simulink model "Proj2_P4_2"  (Simulink 8.6)
settings: Solver=ode45  StartTime=0.0  StopTime=10  MaxStep=0.001  RelTol=1e-3
values from neighbouring files (symbols this model uses):
  fl_rd_0 = fl_rd_rated    [Proj2_IM_IC_rated.m]    (also in Proj2_P1_calc.m = eps)
  fl_rd_0_est2 = fl_rd_rated_est2    [Proj2_P4_S2.m]    (also in Proj2_P4_calc2.m = fl_rd_0; Proj2_P4_calc3.m = fl_rd_0)
  fl_rd_0_est3 = fl_rd_rated    [Proj2_P4_S3.m]    (also in Proj2_P4_calc2.m = fl_rd_0; Proj2_P4_calc3.m = fl_rd_0)
  fl_sd_0 = fl_sd_rated    [Proj2_IM_IC_rated.m]    (also in Proj2_P1_calc.m = 0)
  fl_sq_0 = fl_sq_rated    [Proj2_IM_IC_rated.m]    (also in Proj2_P1_calc.m = 0)
  Isd_rated = real(Is_rated)    [Proj2_IM_IC_rated.m]
  Isd_rated_est2 = real(Is_rated_est2)    [Proj2_P4_S2.m]    (also in Proj2_P4_calc2.m = Isd_rated)
  Isd_rated_est3 = real(Is_rated_est3)    [Proj2_P4_S3.m]    (also in Proj2_P4_calc2.m = Isd_rated)
  Isq_0 = Isq_rated    [Proj2_IM_IC_rated.m]
  Isq_0_est2 = Isq_rated_est2    [Proj2_P4_S2.m]    (also in Proj2_P4_calc2.m = Isq_0; Proj2_P4_calc3.m = Isq_0)
  Isq_0_est3 = Isq_rated_est3    [Proj2_P4_S3.m]    (also in Proj2_P4_calc2.m = Isq_0; Proj2_P4_calc3.m = Isq_0)
  J_eq = 75    [Proj2_IM_parameters.m]
  Ki_i = w_c_i*sqrt(R_s^2+(w_c_i*L_s*sigma)^2) / sqrt(1+wc_Kp_by_Ki_for_i^2)    [Proj2_IM_IC_rated.m]
  Ki_i_est3 = w_c_i*sqrt(R_s^2+(w_c_i*L_s*sigma_est3)^2) / sqrt(1+wc_Kp_by_Ki_for_i_est3^2)    [Proj2_P4_S3.m]    (also in Proj2_P4_calc2.m = Ki_i)
  Ki_s = w_c_s^2*J_eq/(k*sqrt(1+tan(PM_s)^2))    [Proj2_IM_IC_rated.m]
  Ki_s_est2 = w_c_s^2*J_eq/(k_est2*sqrt(1+tan(PM_s)^2))    [Proj2_P4_S2.m]    (also in Proj2_P4_calc2.m = Ki_s)
  Ki_s_est3 = w_c_s^2*J_eq/(k_est3*sqrt(1+tan(PM_s)^2))    [Proj2_P4_S3.m]    (also in Proj2_P4_calc2.m = Ki_s)
  Kp_i = Ki_i * wc_Kp_by_Ki_for_i / w_c_i    [Proj2_IM_IC_rated.m]
  Kp_i_est3 = Ki_i_est3 * wc_Kp_by_Ki_for_i_est3 / w_c_i    [Proj2_P4_S3.m]    (also in Proj2_P4_calc2.m = Kp_i)
  Kp_s = Ki_s * wc_Kp_by_Ki_for_s / w_c_s    [Proj2_IM_IC_rated.m]
  Kp_s_est2 = Ki_s_est2 * wc_Kp_by_Ki_for_s / w_c_s    [Proj2_P4_S2.m]    (also in Proj2_P4_calc2.m = Kp_s)
  Kp_s_est3 = Ki_s_est3 * wc_Kp_by_Ki_for_s / w_c_s    [Proj2_P4_S3.m]    (also in Proj2_P4_calc2.m = Kp_s)
  L_m = X_m /w_syn    (= 0.00152788745368)    [Proj2_IM_parameters.m]
  L_r = L_lr+L_m    (= 0.00161011750761)    [Proj2_IM_parameters.m]
  L_r_est3 = L_lr_est3 + L_m    [Proj2_P4_S3.m]
  L_s = L_ls+L_m    (= 0.00161807525477)    [Proj2_IM_parameters.m]
  p = 6    [Proj2_IM_parameters.m]
  R_s = 1.4*10^-3    (= 0.0014)    [Proj2_IM_parameters.m]
  T_L_rated = T_em_rated    [Proj2_IM_parameters.m]
  tau_r = L_r/R_r    (= 1.62474016914)    [Proj2_IM_parameters.m]
  tau_r_est2 = L_r/R_r_est2    [Proj2_P4_S2.m]
  tau_r_est3 = L_r_est3/R_r    [Proj2_P4_S3.m]
  theta_da_0 = theta_fl_rated_a    [Proj2_IM_IC_rated.m]    (also in Proj2_P1_calc.m = 0)
  theta_dA_0 = theta_fl_rated_a    [Proj2_IM_IC_rated.m]    (also in Proj2_P1_calc.m = 0)
  theta_da_0_est2 = theta_fl_rated_a_est2    [Proj2_P4_S2.m]    (also in Proj2_P4_calc2.m = theta_da_0; Proj2_P4_calc3.m = theta_da_0)
  theta_da_0_est3 = theta_fl_rated_a_est3    [Proj2_P4_S3.m]    (also in Proj2_P4_calc2.m = theta_da_0; Proj2_P4_calc3.m = theta_da_0)
  Vsd_0 = Vsd_rated    [Proj2_IM_IC_rated.m]
  Vsd_prime_0 = Vsd_0 - L_m/L_r*d_fl_rd_0_by_dt + w_syn*sigma*L_s*Isq_0    [Proj2_IM_IC_rated.m]
  Vsq_0 = Vsq_rated    [Proj2_IM_IC_rated.m]
  Vsq_prime_0 = Vsq_0 - w_syn*(L_m/L_r)*fl_rd_0 - w_syn*sigma*L_s*Isd_0    [Proj2_IM_IC_rated.m]
  w_mech_0 = w_mech_rated    [Proj2_IM_IC_rated.m]    (also in Proj2_P1_calc.m = 0)
  w_mech_rated = (1-s)*w_syn/(p/2)    (= 124.407069082)    [Proj2_IM_parameters.m]
(part 2 of 2)

== system Proj2_P4_2/Controllers without Voltage Compensation 1/abc --> dq ==
  a : Inport
  b : Inport  Port=2
  c : Inport  Port=3
  theta_da_est : Inport  Port=4
  Mux1 : Mux
  isd Eq. 3-12 : Fcn  Expr=sqrt(2/3)*(cos(u(4))*u(1)+cos(u(4)-2*pi/3)*u(2)+cos(u(4)-4*pi/3)*u(3))
  isq Eq. 3-12 : Fcn  Expr=-sqrt(2/3)*(sin(u(4))*u(1)+sin(u(4)-2*pi/3)*u(2)+sin(u(4)-4*pi/3)*u(3))
  is_d : Outport
  is_q : Outport  Port=2
  wires:
  theta_da_est/1 -> Mux1/4
  c/1 -> Mux1/3
  b/1 -> Mux1/2
  a/1 -> Mux1/1
  isq Eq. 3-12/1 -> is_q/1
  isd Eq. 3-12/1 -> is_d/1
  Mux1/1 -> isq Eq. 3-12/1, isd Eq. 3-12/1

== system Proj2_P4_2/Controllers without Voltage Compensation 1/dq --> abc  ==
  d : Inport
  q : Inport  Port=2
  theta_da_est : Inport  Port=3
  Mux1 : Mux  Inputs=3
  ia Eq. 3-18 : Fcn  Expr=sqrt(2/3)*(cos(u(3))*u(1)-sin(u(3))*u(2))
  ib Eq. 3-18 : Fcn  Expr=sqrt(2/3)*(cos(u(3)+4*pi/3)*u(1)-sin(u(3)+4*pi/3)*u(2))
  ic Eq. 3-18 : Fcn  Expr=sqrt(2/3)*(cos(u(3)+2*pi/3)*u(1)-sin(u(3)+2*pi/3)*u(2))
  Va : Outport
  Vb : Outport  Port=2
  Vc : Outport  Port=3
  wires:
  ic Eq. 3-18/1 -> Vc/1
  Mux1/1 -> ic Eq. 3-18/1, ib Eq. 3-18/1, ia Eq. 3-18/1
  ib Eq. 3-18/1 -> Vb/1
  d/1 -> Mux1/1
  q/1 -> Mux1/2
  theta_da_est/1 -> Mux1/3
  ia Eq. 3-18/1 -> Va/1

== system Proj2_P4_2/Controllers without Voltage Compensation 2/abc --> dq  ==
  a : Inport
  b : Inport  Port=2
  c : Inport  Port=3
  theta_da_est : Inport  Port=4
  Mux1 : Mux
  isd Eq. 3-12 : Fcn  Expr=sqrt(2/3)*(cos(u(4))*u(1)+cos(u(4)-2*pi/3)*u(2)+cos(u(4)-4*pi/3)*u(3))
  isq Eq. 3-12 : Fcn  Expr=-sqrt(2/3)*(sin(u(4))*u(1)+sin(u(4)-2*pi/3)*u(2)+sin(u(4)-4*pi/3)*u(3))
  is_d : Outport
  is_q : Outport  Port=2
  wires:
  theta_da_est/1 -> Mux1/4
  c/1 -> Mux1/3
  b/1 -> Mux1/2
  a/1 -> Mux1/1
  isq Eq. 3-12/1 -> is_q/1
  isd Eq. 3-12/1 -> is_d/1
  Mux1/1 -> isq Eq. 3-12/1, isd Eq. 3-12/1

== system Proj2_P4_2/Controllers without Voltage Compensation 2/dq --> abc  ==
  d : Inport
  q : Inport  Port=2
  theta_da_est : Inport  Port=3
  Mux1 : Mux  Inputs=3
  ia Eq. 3-18 : Fcn  Expr=sqrt(2/3)*(cos(u(3))*u(1)-sin(u(3))*u(2))
  ib Eq. 3-18 : Fcn  Expr=sqrt(2/3)*(cos(u(3)+4*pi/3)*u(1)-sin(u(3)+4*pi/3)*u(2))
  ic Eq. 3-18 : Fcn  Expr=sqrt(2/3)*(cos(u(3)+2*pi/3)*u(1)-sin(u(3)+2*pi/3)*u(2))
  Va : Outport
  Vb : Outport  Port=2
  Vc : Outport  Port=3
  wires:
  ic Eq. 3-18/1 -> Vc/1
  Mux1/1 -> ic Eq. 3-18/1, ib Eq. 3-18/1, ia Eq. 3-18/1
  ib Eq. 3-18/1 -> Vb/1
  d/1 -> Mux1/1
  q/1 -> Mux1/2
  theta_da_est/1 -> Mux1/3
  ia Eq. 3-18/1 -> Va/1

== system Proj2_P4_2/Controllers without Voltage Compensation 3/abc --> dq  ==
  a : Inport
  b : Inport  Port=2
  c : Inport  Port=3
  theta_da_est : Inport  Port=4
  Mux1 : Mux
  isd Eq. 3-12 : Fcn  Expr=sqrt(2/3)*(cos(u(4))*u(1)+cos(u(4)-2*pi/3)*u(2)+cos(u(4)-4*pi/3)*u(3))
  isq Eq. 3-12 : Fcn  Expr=-sqrt(2/3)*(sin(u(4))*u(1)+sin(u(4)-2*pi/3)*u(2)+sin(u(4)-4*pi/3)*u(3))
  is_d : Outport
  is_q : Outport  Port=2
  wires:
  theta_da_est/1 -> Mux1/4
  c/1 -> Mux1/3
  b/1 -> Mux1/2
  a/1 -> Mux1/1
  isq Eq. 3-12/1 -> is_q/1
  isd Eq. 3-12/1 -> is_d/1
  Mux1/1 -> isq Eq. 3-12/1, isd Eq. 3-12/1

== system Proj2_P4_2/Controllers without Voltage Compensation 3/dq --> abc  ==
  d : Inport
  q : Inport  Port=2
  theta_da_est : Inport  Port=3
  Mux1 : Mux  Inputs=3
  ia Eq. 3-18 : Fcn  Expr=sqrt(2/3)*(cos(u(3))*u(1)-sin(u(3))*u(2))
  ib Eq. 3-18 : Fcn  Expr=sqrt(2/3)*(cos(u(3)+4*pi/3)*u(1)-sin(u(3)+4*pi/3)*u(2))
  ic Eq. 3-18 : Fcn  Expr=sqrt(2/3)*(cos(u(3)+2*pi/3)*u(1)-sin(u(3)+2*pi/3)*u(2))
  Va : Outport
  Vb : Outport  Port=2
  Vc : Outport  Port=3
  wires:
  ic Eq. 3-18/1 -> Vc/1
  Mux1/1 -> ic Eq. 3-18/1, ib Eq. 3-18/1, ia Eq. 3-18/1
  ib Eq. 3-18/1 -> Vb/1
  d/1 -> Mux1/1
  q/1 -> Mux1/2
  theta_da_est/1 -> Mux1/3
  ia Eq. 3-18/1 -> Va/1

== system Proj2_P4_2/Estimated Motor Model/abc --> dq Eq. 3-12 ==
  a : Inport
  b : Inport  Port=2
  c : Inport  Port=3
  theta_da_est : Inport  Port=4
  Mux1 : Mux
  Mux2 : Mux  Inputs=2
  isd Eq. 3-8 : Fcn  Expr=sqrt(2/3)*(cos(u(4))*u(1)+cos(u(4)-2*pi/3)*u(2)+cos(u(4)-4*pi/3)*u(3))
  vsq Eq. 3-8 : Fcn  Expr=-sqrt(2/3)*(sin(u(4))*u(1)+sin(u(4)-2*pi/3)*u(2)+sin(u(4)-4*pi/3)*u(3))
  is_dq : Outport
  wires:
  Mux2/1 -> is_dq/1
  theta_da_est/1 -> Mux1/4
  c/1 -> Mux1/3
  b/1 -> Mux1/2
  a/1 -> Mux1/1
  vsq Eq. 3-8/1 -> Mux2/2
  isd Eq. 3-8/1 -> Mux2/1
  Mux1/1 -> vsq Eq. 3-8/1, isd Eq. 3-8/1

== system Proj2_P4_2/Estimated Motor Model 2/abc --> dq Eq. 3-12 ==
  a : Inport
  b : Inport  Port=2
  c : Inport  Port=3
  theta_da_est : Inport  Port=4
  Mux1 : Mux
  Mux2 : Mux  Inputs=2
  isd Eq. 3-8 : Fcn  Expr=sqrt(2/3)*(cos(u(4))*u(1)+cos(u(4)-2*pi/3)*u(2)+cos(u(4)-4*pi/3)*u(3))
  vsq Eq. 3-8 : Fcn  Expr=-sqrt(2/3)*(sin(u(4))*u(1)+sin(u(4)-2*pi/3)*u(2)+sin(u(4)-4*pi/3)*u(3))
  is_dq : Outport
  wires:
  Mux2/1 -> is_dq/1
  theta_da_est/1 -> Mux1/4
  c/1 -> Mux1/3
  b/1 -> Mux1/2
  a/1 -> Mux1/1
  vsq Eq. 3-8/1 -> Mux2/2
  isd Eq. 3-8/1 -> Mux2/1
  Mux1/1 -> vsq Eq. 3-8/1, isd Eq. 3-8/1

== system Proj2_P4_2/Estimated Motor Model 3/abc --> dq Eq. 3-12 ==
  a : Inport
  b : Inport  Port=2
  c : Inport  Port=3
  theta_da_est : Inport  Port=4
  Mux1 : Mux
  Mux2 : Mux  Inputs=2
  isd Eq. 3-8 : Fcn  Expr=sqrt(2/3)*(cos(u(4))*u(1)+cos(u(4)-2*pi/3)*u(2)+cos(u(4)-4*pi/3)*u(3))
  vsq Eq. 3-8 : Fcn  Expr=-sqrt(2/3)*(sin(u(4))*u(1)+sin(u(4)-2*pi/3)*u(2)+sin(u(4)-4*pi/3)*u(3))
  is_dq : Outport
  wires:
  Mux2/1 -> is_dq/1
  theta_da_est/1 -> Mux1/4
  c/1 -> Mux1/3
  b/1 -> Mux1/2
  a/1 -> Mux1/1
  vsq Eq. 3-8/1 -> Mux2/2
  isd Eq. 3-8/1 -> Mux2/1
  Mux1/1 -> vsq Eq. 3-8/1, isd Eq. 3-8/1
